simulink library "LIB_TF_G_12_StepControl"  (Simulink 8.6)
settings: Solver=ode45  StartTime=0.0  StopTime=10.0  RelTol=1e-3
PreLoadFcn:
  | if exist('tl_preloadfcn','file'), tl_preloadfcn(gcs,402); end
PostLoadFcn:
  | if exist('tl_postloadfcn','file'), tl_postloadfcn(gcs,402); end
undefined symbols (not defined in the file): ddv, u2, u3
libraries: tllib x4, LIB_TF_G_12_StepControl x1
(part 5 of 7)

== system LIB_TF_G_12_StepControl/TF_G_12_ManageEndingStep/Step execution in progress/ManageBeltPayOutAbortion/Belt Payout Abortion Opt Activated ==
  note: Belt Payout Interruption
  bBeltPayOutAbortion2 : Inport  RequirementInfo={} %GIDa_c23c1519_ce77_4f0e_84e0_58e9ce6e7015
  bBeltPayOutAbortion1 : Inport  RequirementInfo={} %GIDa_65d5ef8b_71e9_4e52_9127_813aec9379ea  Port=2
  u16BeltPayOutFiltered_mm : Inport  RequirementInfo={} %GIDa_03e05a97_4a46_4a00_a943_78f19d364a7f  Port=3
  Action Port : ActionPort  RequirementInfo={} %GIDa_ed5b74e4_286f_4c4b_a0da_10247e3268a9
  Constant3 : Constant  RequirementInfo={} %GIDa_df278d9b_a5ca_4067_b82a_a721af7a99c6  Value=ddv('BFE_Config_Data/CAL_KU16_BELT_PAYOUT_ABORTION_THRS1')  OutDataTypeStr=uint16  mask(TL_Constant){data={'output',{'variable','BFE_Config_Data/CAL_KU16_BELT_PAYOUT_ABORTION_THRS1'},'autoscaling',{'mode',2,'scalingvalid',1},'date',735951.66847480321}}
      settings: CopyFcn=if exist('tl_reset_reviewflag','file')==2,tl_reset_reviewflag(gcbh);end  DeleteFcn=if exist('delete_tlblock','file')==2,delete_tlblock(gcbh);end  NameChangeFcn=if exist('rename_tlblock','file')==2,rename_tlblock(gcbh);end  OpenFcn=if exist('tl_open_blockdlg','file')==2,tl_open_blockdlg(gcbh);else,open_system(gcbh,'parameter');end
      mask Help: eval(['if exist(''tl_online_help'',''file'') == 2, tl_online_help(''Topic'',''TL_Constant''),else, web([''jar:file:///'',matlabroot,''/help/toolbox/simulink/help.jar!/slref/' lower(get_param(gcbh,'Blocktype')) '.html''], ''-helpbrowser''),end'])
      mask Display: plot([-0.05, 1.05, NaN, -0.05, 1.05],[.01, .01, NaN, .99, .99])
  Constant5 : Constant  RequirementInfo={} %GIDa_6b8f2a3b_36a6_49af_a030_774c3046518c  Value=ddv('BFE_Config_Data/CAL_KU16_BELT_PAYOUT_ABORTION_THRS2')  OutDataTypeStr=uint16  mask(TL_Constant){data={'output',{'variable','BFE_Config_Data/CAL_KU16_BELT_PAYOUT_ABORTION_THRS2'},'autoscaling',{'mode',2,'scalingvalid',1},'date',735951.66847444442}}
      settings: CopyFcn=if exist('tl_reset_reviewflag','file')==2,tl_reset_reviewflag(gcbh);end  DeleteFcn=if exist('delete_tlblock','file')==2,delete_tlblock(gcbh);end  NameChangeFcn=if exist('rename_tlblock','file')==2,rename_tlblock(gcbh);end  OpenFcn=if exist('tl_open_blockdlg','file')==2,tl_open_blockdlg(gcbh);else,open_system(gcbh,'parameter');end
      mask Help: eval(['if exist(''tl_online_help'',''file'') == 2, tl_online_help(''Topic'',''TL_Constant''),else, web([''jar:file:///'',matlabroot,''/help/toolbox/simulink/help.jar!/slref/' lower(get_param(gcbh,'Blocktype')) '.html''], ''-helpbrowser''),end'])
      mask Display: plot([-0.05, 1.05, NaN, -0.05, 1.05],[.01, .01, NaN, .99, .99])
  Relational Operator1 : RelationalOperator  RequirementInfo={} %GIDa_2e279048_a574_4730_af74_afcb5488e17b  Operator=<=  OutDataTypeStr=boolean  mask(TL_RelationalOperator){data={'date',735951.6684740741}}
      settings: DeleteFcn=if exist('delete_tlblock','file')==2,delete_tlblock(gcbh);end  NameChangeFcn=if exist('rename_tlblock','file')==2,rename_tlblock(gcbh);end  OpenFcn=if exist('tl_open_blockdlg','file')==2,tl_open_blockdlg(gcbh);else,open_system(gcbh,'parameter');end
      mask Help: eval(['if exist(''tl_online_help'',''file'') == 2, tl_online_help(''Topic'',''TL_RelationalOperator''),else, web([''jar:file:///'',matlabroot,''/help/toolbox/simulink/help.jar!/slref/' lower(get_param(gcbh,'Blocktype')) '.html''], ''-helpbrowser''),end'])
      mask Display: plot([-0.05, 1.05, NaN, -0.05, 1.05],[.01, .01, NaN, .99, .99])
  Relational Operator2 : RelationalOperator  RequirementInfo={} %GIDa_1c9f918a_1d2a_4c1b_b35b_2dc0061f631d  OutDataTypeStr=boolean  mask(TL_RelationalOperator){data={'date',735951.66847383103}}
      settings: DeleteFcn=if exist('delete_tlblock','file')==2,delete_tlblock(gcbh);end  NameChangeFcn=if exist('rename_tlblock','file')==2,rename_tlblock(gcbh);end  OpenFcn=if exist('tl_open_blockdlg','file')==2,tl_open_blockdlg(gcbh);else,open_system(gcbh,'parameter');end
      mask Help: eval(['if exist(''tl_online_help'',''file'') == 2, tl_online_help(''Topic'',''TL_RelationalOperator''),else, web([''jar:file:///'',matlabroot,''/help/toolbox/simulink/help.jar!/slref/' lower(get_param(gcbh,'Blocktype')) '.html''], ''-helpbrowser''),end'])
      mask Display: plot([-0.05, 1.05, NaN, -0.05, 1.05],[.01, .01, NaN, .99, .99])
  anyBeltPayOutEvent : Logic  RequirementInfo="{'linktype_rmi_doors' '0000eac7 (/106886 BMW BMW L7 EL ECU PP R-EVAS-EMA_Phase_0/30_PRO_Requirements/Specification/05 Product Requirements/01 Main Functions/04_MF-04_To_Park_The_Belt_When_It_Is_Not_Fastened)' '#180' 'true' '2.3.2.1.1.0-19 Step 3:\t Abort step 3 (and go to Step 4) as soon as the belt ' ' ' ; 'linktype_rmi_doors' '0000eac7 (/106886 BMW BMW L7 EL ECU PP R-EVAS-EMA_Phase_0/30_PRO_Requirements/Specification/05 Product Requirements/01 Main Functions/04_MF-04_To_Park_The_Belt_When_It_Is_Not_Fastened)' '#186' 'true' '2.3.2.1.1.0-24 Step 5:\t Abort step 5 (and go to Step 6) as soon as the belt ' ' ' ; 'linktype_rmi_doors' '0000eac7 (/106886 BMW BMW L7 EL ECU PP R-EVAS-EMA_Phase_0/30_PRO_Requirements/Specification/05 Product Requirements/01 Main Functions/04_MF-04_To_Park_The_Belt_When_It_Is_Not_Fastened)' '#219' 'true' '2.3.2.2.1.0-19 Step 3:\t Abort step 3 (and go to Step 4) as soon as the belt ' '' ; 'linktype_rmi_doors' '0000eac7 (/106886 BMW BMW L7 EL ECU PP R-EVAS-EMA_Phase_0/30_PRO_Requirements/Specification/05 Product Requirements/01 Main Functions/04_MF-04_To_Park_The_Belt_When_It_Is_Not_Fastened)' '#224' 'true' '2.3.2.2.1.0-24 Step 5:\t Abort step 5 (and go to Step 6) as soon as the belt ' '' ; 'linktype_rmi_doors' '0000eac7 (/106886 BMW BMW L7 EL ECU PP R-EVAS-EMA_Phase_0/30_PRO_Requirements/Specification/05 Product Requirements/01 Main Functions/04_MF-04_To_Park_The_Belt_When_It_Is_Not_Fastened)' '#466' 'true' '2.4.4.2.1.2 Belt Payout' ' ' ; 'linktype_rmi_doors' '0000eac7 (/106886 BMW BMW L7 EL ECU PP R-EVAS-EMA_Phase_0/30_PRO_Requirements/Specification/05 Product Requirements/01 Main Functions/04_MF-04_To_Park_The_Belt_When_It_Is_Not_Fastened)' '#829' 'true' '2.4.4.2.1.2.1 High threshold' ' ' ; 'linktype_rmi_doors' '0000eac7 (/106886 BMW BMW L7 EL ECU PP R-EVAS-EMA_Phase_0/30_PRO_Requirements/Specification/05 Product Requirements/01 Main Functions/04_MF-04_To_Park_The_Belt_When_It_Is_Not_Fastened)' '#831' 'true' '2.4.4.2.1.2.1.0-1 Definition: Used to specify the minimum value of the belt pos' '' ; 'linktype_rmi_doors' '0000eac7 (/106886 BMW BMW L7 EL ECU PP R-EVAS-EMA_Phase_0/30_PRO_Requirements/Specification/05 Product Requirements/01 Main Functions/04_MF-04_To_Park_The_Belt_When_It_Is_Not_Fastened)' '#832' 'true' '2.4.4.2.1.2.1.0-2 Name: u16NvmHiBeltPayoutAbortThrs' ' ' ; 'linktype_rmi_doors' '0000eac7 (/106886 BMW BMW L7 EL ECU PP R-EVAS-EMA_Phase_0/30_PRO_Requirements/Specification/05 Product Requirements/01 Main Functions/04_MF-04_To_Park_The_Belt_When_It_Is_Not_Fastened)' '#833' 'true' '2.4.4.2.1.2.1.0-3 Type: SAFETY SOFTWARE' '' ; 'linktype_rmi_doors' '0000eac7 (/106886 BMW BMW L7 EL ECU PP R-EVAS-EMA_Phase_0/30_PRO_Requirements/Specification/05 Product Requirements/01 Main Functions/04_MF-04_To_Park_The_Belt_When_It_Is_Not_Fastened)' '#834' 'true' '2.4.4.2.1.2.1.0-4 Size: 2 bytes' '' ; 'linktype_rmi_doors' '0000eac7 (/106886 BMW BMW L7 EL ECU PP R-EVAS-EMA_Phase_0/30_PRO_Requirements/Specification/05 Product Requirements/01 Main Functions/04_MF-04_To_Park_The_Belt_When_It_Is_Not_Fastened)' '#835' 'true' '2.4.4.2.1.2.1.0-5 Scaling: 1LSB = 1mm' '' ; 'linktype_rmi_doors' '0000eac7 (/106886 BMW BMW L7 EL ECU PP R-EVAS-EMA_Phase_0/30_PRO_Requirements/Specification/05 Product Requirements/01 Main Functions/04_MF-04_To_Park_The_Belt_When_It_Is_Not_Fastened)' '#836' 'true' '2.4.4.2.1.2.1.0-6 Constraints: Unsigned full range = [0 ; 65535] = [0mm ; 65535' '' ; 'linktype_rmi_doors' '0000eac7 (/106886 BMW BMW L7 EL ECU PP R-EVAS-EMA_Phase_0/30_PRO_Requirements/Specification/05 Product Requirements/01 Main Functions/04_MF-04_To_Park_The_Belt_When_It_Is_Not_Fastened)' '#837' 'true' '2.4.4.2.1.2.1.0-7 Default value: 0x02EE = 750mm' '' ; 'linktype_rmi_doors' '0000eac7 (/106886 BMW BMW L7 EL ECU PP R-EVAS-EMA_Phase_0/30_PRO_Requirements/Specification/05 Product Requirements/01 Main Functions/04_MF-04_To_Park_The_Belt_When_It_Is_Not_Fastened)' '#838' 'true' '2.4.4.2.1.2.1.0-8 Access in normal mode (out of diagnosis session): READ only' '' ; 'linktype_rmi_doors' '0000eac7 (/106886 BMW BMW L7 EL ECU PP R-EVAS-EMA_Phase_0/30_PRO_Requirements/Specification/05 Product Requirements/01 Main Functions/04_MF-04_To_Park_The_Belt_When_It_Is_Not_Fastened)' '#830' 'true' '2.4.4.2.1.2.2 Low threshold' ' ' ; 'linktype_rmi_doors' '0000eac7 (/106886 BMW BMW L7 EL ECU PP R-EVAS-EMA_Phase_0/30_PRO_Requirements/Specification/05 Product Requirements/01 Main Functions/04_MF-04_To_Park_The_Belt_When_It_Is_Not_Fastened)' '#839' 'true' '2.4.4.2.1.2.2.0-1 Definition: Used to specify the minimum value of the belt pos' '' ; 'linktype_rmi_doors' '0000eac7 (/106886 BMW BMW L7 EL ECU PP R-EVAS-EMA_Phase_0/30_PRO_Requirements/Specification/05 Product Requirements/01 Main Functions/04_MF-04_To_Park_The_Belt_When_It_Is_Not_Fastened)' '#840' 'true' '2.4.4.2.1.2.2.0-2 Name: u16NvmLowBeltPayoutAbortThrs' ' ' ; 'linktype_rmi_doors' '0000eac7 (/106886 BMW BMW L7 EL ECU PP R-EVAS-EMA_Phase_0/30_PRO_Requirements/Specification/05 Product Requirements/01 Main Functions/04_MF-04_To_Park_The_Belt_When_It_Is_Not_Fastened)' '#841' 'true' '2.4.4.2.1.2.2.0-3 Type: SAFETY SOFTWARE' '' ; 'linktype_rmi_doors' '0000eac7 (/106886 BMW BMW L7 EL ECU PP R-EVAS-EMA_Phase_0/30_PRO_Requirements/Specification/05 Product Requirements/01 Main Functions/04_MF-04_To_Park_The_Belt_When_It_Is_Not_Fastened)' '#842' 'true' '2.4.4.2.1.2.2.0-4 Size: 2 bytes' '' ; 'linktype_rmi_doors' '0000eac7 (/106886 BMW BMW L7 EL ECU PP R-EVAS-EMA_Phase_0/30_PRO_Requirements/Specification/05 Product Requirements/01 Main Functions/04_MF-04_To_Park_The_Belt_When_It_Is_Not_Fastened)' '#843' 'true' '2.4.4.2.1.2.2.0-5 Scaling: 1LSB = 1mm' '' ; 'linktype_rmi_doors' '0000eac7 (/106886 BMW BMW L7 EL ECU PP R-EVAS-EMA_Phase_0/30_PRO_Requirements/Specification/05 Product Requirements/01 Main Functions/04_MF-04_To_Park_The_Belt_When_It_Is_Not_Fastened)' '#844' 'true' '2.4.4.2.1.2.2.0-6 Constraints: Unsigned full range = [0 ; 65535] = [0mm ; 65535' '' ; 'linktype_rmi_doors' '0000eac7 (/106886 BMW BMW L7 EL ECU PP R-EVAS-EMA_Phase_0/30_PRO_Requirements/Specification/05 Product Requirements/01 Main Functions/04_MF-04_To_Park_The_Belt_When_It_Is_Not_Fastened)' '#845' 'true' '2.4.4.2.1.2.2.0-7 Default value: 0x012C = 300mm' '' ; 'linktype_rmi_doors' '0000eac7 (/106886 BMW BMW L7 EL ECU PP R-EVAS-EMA_Phase_0/30_PRO_Requirements/Specification/05 Product Requirements/01 Main Functions/04_MF-04_To_Park_The_Belt_When_It_Is_Not_Fastened)' '#846' 'true' '2.4.4.2.1.2.2.0-8 Access in normal mode (out of diagnosis session): READ only' ' ' } %GIDa_a8192212_6ba7_426f_b05f_69b939d358c2"  Operator=OR  AllPortsSameDT=off  OutDataTypeStr=boolean  mask(TL_LogicalOperator){data={'date',735951.66847358795}}
      settings: DeleteFcn=if exist('delete_tlblock','file')==2,delete_tlblock(gcbh);end  NameChangeFcn=if exist('rename_tlblock','file')==2,rename_tlblock(gcbh);end  OpenFcn=if exist('tl_open_blockdlg','file')==2,tl_open_blockdlg(gcbh);else,open_system(gcbh,'parameter');end
      mask Help: eval(['if exist(''tl_online_help'',''file'') == 2, tl_online_help(''Topic'',''TL_LogicalOperator''),else, web([''jar:file:///'',matlabroot,''/help/toolbox/simulink/help.jar!/slref/' lower(get_param(gcbh,'Blocktype')) '.html''], ''-helpbrowser''),end'])
      mask Display: plot([-0.05, 1.05, NaN, -0.05, 1.05],[.01, .01, NaN, .99, .99])
  bBeltPayoutStepOptionExclusiveSet : Logic  RequirementInfo={} %GIDa_2a375b25_5cfa_4ca7_9be7_2ef03136cf89  Operator=XOR  AllPortsSameDT=off  OutDataTypeStr=boolean  mask(TL_LogicalOperator){data={'comment',{'text',['COD_BFE_00001' char(10) 'PO bits are defined for the "Belt PayOut Controlled" constraint under the following configuration:' char(10) '- 00 : "Belt PayOut controlled" constraint is not used' char(10) '- 01 : Low threshold (u16NvmLowBeltPayoutAbortThrs) is used' char(10) '- 10 : High threshold (u16NvmHiBeltPayoutAbortThrs) is used' char(10) '[COVERS : PRO_MF4_968]']},'output',{'name','$B'},'date',735951.66847333335}}
      settings: DeleteFcn=if exist('delete_tlblock','file')==2,delete_tlblock(gcbh);end  NameChangeFcn=if exist('rename_tlblock','file')==2,rename_tlblock(gcbh);end  OpenFcn=if exist('tl_open_blockdlg','file')==2,tl_open_blockdlg(gcbh);else,open_system(gcbh,'parameter');end
      mask Help: eval(['if exist(''tl_online_help'',''file'') == 2, tl_online_help(''Topic'',''TL_LogicalOperator''),else, web([''jar:file:///'',matlabroot,''/help/toolbox/simulink/help.jar!/slref/' lower(get_param(gcbh,'Blocktype')) '.html''], ''-helpbrowser''),end'])
      mask Display: plot([-0.05, 1.05, NaN, -0.05, 1.05],[.01, .01, NaN, .99, .99])
  u16NvmBeltPayoutAbortThrs1_Satisfy : Logic  RequirementInfo={} %GIDa_b2515d3c_dd19_480b_875b_9924ba5bbf92  Inputs=3  AllPortsSameDT=off  OutDataTypeStr=boolean  mask(TL_LogicalOperator){data={'date',735951.66847305559}}
      settings: DeleteFcn=if exist('delete_tlblock','file')==2,delete_tlblock(gcbh);end  NameChangeFcn=if exist('rename_tlblock','file')==2,rename_tlblock(gcbh);end  OpenFcn=if exist('tl_open_blockdlg','file')==2,tl_open_blockdlg(gcbh);else,open_system(gcbh,'parameter');end
      mask Help: eval(['if exist(''tl_online_help'',''file'') == 2, tl_online_help(''Topic'',''TL_LogicalOperator''),else, web([''jar:file:///'',matlabroot,''/help/toolbox/simulink/help.jar!/slref/' lower(get_param(gcbh,'Blocktype')) '.html''], ''-helpbrowser''),end'])
      mask Display: plot([-0.05, 1.05, NaN, -0.05, 1.05],[.01, .01, NaN, .99, .99])
  u16NvmBeltPayoutAbortThrs2_Satisfy : Logic  RequirementInfo={} %GIDa_f1047f13_8326_4e3c_a34e_0d6ae5728ff1  Inputs=3  AllPortsSameDT=off  OutDataTypeStr=boolean  mask(TL_LogicalOperator){data={'date',735951.66847275465}}
      settings: DeleteFcn=if exist('delete_tlblock','file')==2,delete_tlblock(gcbh);end  NameChangeFcn=if exist('rename_tlblock','file')==2,rename_tlblock(gcbh);end  OpenFcn=if exist('tl_open_blockdlg','file')==2,tl_open_blockdlg(gcbh);else,open_system(gcbh,'parameter');end
      mask Help: eval(['if exist(''tl_online_help'',''file'') == 2, tl_online_help(''Topic'',''TL_LogicalOperator''),else, web([''jar:file:///'',matlabroot,''/help/toolbox/simulink/help.jar!/slref/' lower(get_param(gcbh,'Blocktype')) '.html''], ''-helpbrowser''),end'])
      mask Display: plot([-0.05, 1.05, NaN, -0.05, 1.05],[.01, .01, NaN, .99, .99])
  bShallStepContinue : Outport  RequirementInfo={} %GIDa_64a204de_75df_4cc5_b6bd_1c3b809efabe
  wires:
  Relational Operator1/1 -> u16NvmBeltPayoutAbortThrs1_Satisfy/3
  Constant3/1 -> Relational Operator1/2
  Constant5/1 -> Relational Operator2/1
  Relational Operator2/1 -> u16NvmBeltPayoutAbortThrs2_Satisfy/1
  bBeltPayOutAbortion2/1 -> u16NvmBeltPayoutAbortThrs2_Satisfy/2, bBeltPayoutStepOptionExclusiveSet/1
  u16NvmBeltPayoutAbortThrs2_Satisfy/1 -> anyBeltPayOutEvent/1
  u16NvmBeltPayoutAbortThrs1_Satisfy/1 -> anyBeltPayOutEvent/2
  anyBeltPayOutEvent/1 -> bShallStepContinue/1
  u16BeltPayOutFiltered_mm/1 -> Relational Operator2/2, Relational Operator1/1
  bBeltPayoutStepOptionExclusiveSet/1 -> u16NvmBeltPayoutAbortThrs2_Satisfy/3, u16NvmBeltPayoutAbortThrs1_Satisfy/1
  bBeltPayOutAbortion1/1 -> u16NvmBeltPayoutAbortThrs1_Satisfy/2, bBeltPayoutStepOptionExclusiveSet/2

== system LIB_TF_G_12_StepControl/TF_G_12_ManageEndingStep/Step execution in progress/ManageBeltPayOutAbortion/Belt Payout Abortion Opt Deactivated ==
  Action Port : ActionPort  RequirementInfo={} %GIDa_c6f90e3b_f66f_4145_a0bd_dd5fd3e7edbc
  KB_FALSE : Constant  RequirementInfo={} %GIDa_fd22fdc3_6d5e_4ed9_8abf_b1b892869fac  Value=ddv('BFE/KB_FALSE')  OutDataTypeStr=boolean  SampleTime=-1  mask(TL_Constant){data={'output',{'variable','BFE/KB_FALSE'},'date',735951.66847248841}}
      settings: CopyFcn=if exist('tl_reset_reviewflag','file')==2,tl_reset_reviewflag(gcbh);end  DeleteFcn=if exist('delete_tlblock','file')==2,delete_tlblock(gcbh);end  NameChangeFcn=if exist('rename_tlblock','file')==2,rename_tlblock(gcbh);end  OpenFcn=if exist('tl_open_blockdlg','file')==2,tl_open_blockdlg(gcbh);else,open_system(gcbh,'parameter');end
      mask Help: eval(['if exist(''tl_online_help'',''file'') == 2, tl_online_help(''Topic'',''TL_Constant''),else, web([''jar:file:///'',matlabroot,''/help/toolbox/simulink/help.jar!/slref/' lower(get_param(gcbh,'Blocktype')) '.html''], ''-helpbrowser''),end'])
      mask Display: plot([-0.05, 1.05, NaN, -0.05, 1.05],[.01, .01, NaN, .99, .99])
  bShallStepContinue : Outport  RequirementInfo={} %GIDa_519f0a92_0f2a_43d0_80ad_a80812805cc2
  wires:
  KB_FALSE/1 -> bShallStepContinue/1

== system LIB_TF_G_12_StepControl/TF_G_12_ManageEndingStep/Step execution in progress/ManageMotorBlocked (Motor OverCurrent)/Motor Blocked Opt Activated ==
  u32MotorCurrent : Inport  RequirementInfo={} %GIDa_35077fa2_8525_40e9_ae14_395478e9e03d
  u16Temperature : Inport  RequirementInfo={} %GIDa_61ac1d77_d44d_43cd_babc_899375823a81  Port=2
  s16MotorPower : Inport  RequirementInfo={} %GIDa_1fed8ada_d606_4b4d_92f8_f6734bb26c11  Port=3
  u16BatteryVoltage : Inport  RequirementInfo={} %GIDa_ddfb933f_dae9_4570_b46d_68e419ca580a  Port=4
  bMotorBlockedControlled : Inport  RequirementInfo={} %GIDa_ae8f7be4_9352_48c1_9f9d_6020105d65ee  Port=5
  e_StepValidity Internal Status : Inport  RequirementInfo={} %GIDa_ddfb933f_dae9_4570_b46d_68e419ca580a  Port=6
  Action Port : ActionPort  RequirementInfo={} %GIDa_87bb87ed_56e9_449a_a862_c49058b79593
  If : If  RequirementInfo={} %GIDa_8d0784e2_3fab_4adf_9f81_7b4d294112bc  IfExpression=~u1
  If Action Subsystem : Subsystem  RequirementInfo={} %GIDa_865aa8e5_6704_479c_ad50_26c0c78900e7  TreatAsAtomicUnit=on
  If Action Subsystem1 : Subsystem  RequirementInfo={} %GIDa_8c5d38af_f00b_4300_b53e_cc8f71a37b7d  TreatAsAtomicUnit=on
  Merge : Merge  RequirementInfo={} %GIDa_e9bcc02d_e27f_4329_9329_51a7ee440049  mask(TL_Merge){data={'date',735951.66845872684}}
      settings: CopyFcn=if exist('tl_reset_reviewflag','file')==2,tl_reset_reviewflag(gcbh);end  DeleteFcn=if exist('delete_tlblock','file')==2,delete_tlblock(gcbh);end  NameChangeFcn=if exist('rename_tlblock','file')==2,rename_tlblock(gcbh);end  OpenFcn=if exist('tl_open_blockdlg','file')==2,tl_open_blockdlg(gcbh);else,open_system(gcbh,'parameter');end
      mask Help: eval(['if exist(''tl_online_help'',''file'') == 2, tl_online_help(''Topic'',''TL_Merge''),else, web([''jar:file:///'',matlabroot,''/help/toolbox/simulink/help.jar!/slref/' lower(get_param(gcbh,'Blocktype')) '.html''], ''-helpbrowser''),end'])
      mask Display: plot([-0.05, 1.05, NaN, -0.05, 1.05],[.01, .01, NaN, .99, .99])
  bInterruptStep : Outport  RequirementInfo={} %GIDa_c2568f75_19fb_49aa_9a96_6839ea089117
  wires:
  If/1 -> If Action Subsystem/Action
  bMotorBlockedControlled/1 -> If/1
  If/2 -> If Action Subsystem1/Action
  u32MotorCurrent/1 -> If Action Subsystem1/1(u32MotorCurrent)
  u16Temperature/1 -> If Action Subsystem1/2(u16Temperature)
  s16MotorPower/1 -> If Action Subsystem1/3(s16MotorPower)
  u16BatteryVoltage/1 -> If Action Subsystem1/4(u16BatteryVoltage)
  If Action Subsystem/1(bInterruptStep) -> Merge/1
  If Action Subsystem1/1(bInterruptStep) -> Merge/2
  Merge/1 -> bInterruptStep/1
  e_StepValidity Internal Status/1 -> If Action Subsystem1/5(e_StepValidity)

== system LIB_TF_G_12_StepControl/TF_G_12_ManageEndingStep/Step execution in progress/ManageMotorBlocked (Motor OverCurrent)/Motor Blocked Opt Deactivated ==
  Action Port : ActionPort  RequirementInfo={} %GIDa_c927e320_c65f_4372_9111_160f402852fa
  KB_FALSE : Constant  RequirementInfo={} %GIDa_fd272ef1_75ca_43bb_9878_25ed4256448c  Value=ddv('BFE/KB_FALSE')  OutDataTypeStr=boolean  SampleTime=-1  mask(TL_Constant){data={'output',{'variable','BFE/KB_FALSE'},'date',735951.66845836805}}
      settings: CopyFcn=if exist('tl_reset_reviewflag','file')==2,tl_reset_reviewflag(gcbh);end  DeleteFcn=if exist('delete_tlblock','file')==2,delete_tlblock(gcbh);end  NameChangeFcn=if exist('rename_tlblock','file')==2,rename_tlblock(gcbh);end  OpenFcn=if exist('tl_open_blockdlg','file')==2,tl_open_blockdlg(gcbh);else,open_system(gcbh,'parameter');end
      mask Help: eval(['if exist(''tl_online_help'',''file'') == 2, tl_online_help(''Topic'',''TL_Constant''),else, web([''jar:file:///'',matlabroot,''/help/toolbox/simulink/help.jar!/slref/' lower(get_param(gcbh,'Blocktype')) '.html''], ''-helpbrowser''),end'])
      mask Display: plot([-0.05, 1.05, NaN, -0.05, 1.05],[.01, .01, NaN, .99, .99])
  bInterruptStep : Outport  RequirementInfo={} %GIDa_46abf0d2_941a_4ccb_a280_e17c4bf6b063  InitialOutput=0
  wires:
  KB_FALSE/1 -> bInterruptStep/1

== system LIB_TF_G_12_StepControl/TF_G_12_ManageEndingStep/Step execution in progress/ManageTriggOff (end of holding steps)/TriggOff Opt Activated ==
  bTriggOffControlled : Inport  RequirementInfo={} %GIDa_cf12ec5b_9854_423e_a44e_6913c9bc66ab
  bIsNoMoreTensioningSituation : Inport  RequirementInfo={} %GIDa_3becb22c_9d79_4d7f_b005_4e906a452248  Port=2
  Action Port : ActionPort  RequirementInfo={} %GIDa_3b114ffe_8f83_495a_875f_317d4f567315
  B_TRUE : Constant  RequirementInfo={} %GIDa_b118b147_97b3_4247_834a_d341a382e0c8  Value=ddv('RTE_Define/KU8_TRUE')  OutDataTypeStr=uint8  SampleTime=-1  mask(TL_Constant){data={'output',{'variable','RTE_Define/KU8_TRUE'},'date',735951.66845699074}}
      settings: CopyFcn=if exist('tl_reset_reviewflag','file')==2,tl_reset_reviewflag(gcbh);end  DeleteFcn=if exist('delete_tlblock','file')==2,delete_tlblock(gcbh);end  NameChangeFcn=if exist('rename_tlblock','file')==2,rename_tlblock(gcbh);end  OpenFcn=if exist('tl_open_blockdlg','file')==2,tl_open_blockdlg(gcbh);else,open_system(gcbh,'parameter');end
      mask Help: eval(['if exist(''tl_online_help'',''file'') == 2, tl_online_help(''Topic'',''TL_Constant''),else, web([''jar:file:///'',matlabroot,''/help/toolbox/simulink/help.jar!/slref/' lower(get_param(gcbh,'Blocktype')) '.html''], ''-helpbrowser''),end'])
      mask Display: plot([-0.05, 1.05, NaN, -0.05, 1.05],[.01, .01, NaN, .99, .99])
  ManageTriggOff : Logic  RequirementInfo={} %GIDa_5649dccd_f0a5_450a_b266_b3777bd95ecf  AllPortsSameDT=off  OutDataTypeStr=boolean  mask(TL_LogicalOperator){data={'date',735951.66845665511}}
      settings: DeleteFcn=if exist('delete_tlblock','file')==2,delete_tlblock(gcbh);end  NameChangeFcn=if exist('rename_tlblock','file')==2,rename_tlblock(gcbh);end  OpenFcn=if exist('tl_open_blockdlg','file')==2,tl_open_blockdlg(gcbh);else,open_system(gcbh,'parameter');end
      mask Help: eval(['if exist(''tl_online_help'',''file'') == 2, tl_online_help(''Topic'',''TL_LogicalOperator''),else, web([''jar:file:///'',matlabroot,''/help/toolbox/simulink/help.jar!/slref/' lower(get_param(gcbh,'Blocktype')) '.html''], ''-helpbrowser''),end'])
      mask Display: plot([-0.05, 1.05, NaN, -0.05, 1.05],[.01, .01, NaN, .99, .99])
  RelationalOperator_bAccelerationLow : RelationalOperator  RequirementInfo={} %GIDa_26f27c81_779d_4171_a911_7f443c701b00  Operator===  OutDataTypeStr=boolean  mask(TL_RelationalOperator){data={'date',735951.66845641204}}
      settings: DeleteFcn=if exist('delete_tlblock','file')==2,delete_tlblock(gcbh);end  NameChangeFcn=if exist('rename_tlblock','file')==2,rename_tlblock(gcbh);end  OpenFcn=if exist('tl_open_blockdlg','file')==2,tl_open_blockdlg(gcbh);else,open_system(gcbh,'parameter');end
      mask Help: eval(['if exist(''tl_online_help'',''file'') == 2, tl_online_help(''Topic'',''TL_RelationalOperator''),else, web([''jar:file:///'',matlabroot,''/help/toolbox/simulink/help.jar!/slref/' lower(get_param(gcbh,'Blocktype')) '.html''], ''-helpbrowser''),end'])
      mask Display: plot([-0.05, 1.05, NaN, -0.05, 1.05],[.01, .01, NaN, .99, .99])
  bInterruptStep : Outport  RequirementInfo={} %GIDa_b6b92ec6_f112_4233_b8e9_8b9c41e8818c
  wires:
  RelationalOperator_bAccelerationLow/1 -> ManageTriggOff/2
  ManageTriggOff/1 -> bInterruptStep/1
  bTriggOffControlled/1 -> ManageTriggOff/1
  B_TRUE/1 -> RelationalOperator_bAccelerationLow/1
  bIsNoMoreTensioningSituation/1 -> RelationalOperator_bAccelerationLow/2

== system LIB_TF_G_12_StepControl/TF_G_12_ManageEndingStep/Step execution in progress/ManageTriggOff (end of holding steps)/TriggOff Opt Deactivated ==
  Action Port : ActionPort  RequirementInfo={} %GIDa_16121e16_5dbd_4791_9fa3_71739519c178
  KB_FALSE : Constant  RequirementInfo={} %GIDa_5f17e89d_8651_44bc_898e_efb4f55be7d3  Value=ddv('BFE/KB_FALSE')  OutDataTypeStr=boolean  SampleTime=-1  mask(TL_Constant){data={'output',{'variable','BFE/KB_FALSE'},'date',735951.66845615744}}
      settings: CopyFcn=if exist('tl_reset_reviewflag','file')==2,tl_reset_reviewflag(gcbh);end  DeleteFcn=if exist('delete_tlblock','file')==2,delete_tlblock(gcbh);end  NameChangeFcn=if exist('rename_tlblock','file')==2,rename_tlblock(gcbh);end  OpenFcn=if exist('tl_open_blockdlg','file')==2,tl_open_blockdlg(gcbh);else,open_system(gcbh,'parameter');end
      mask Help: eval(['if exist(''tl_online_help'',''file'') == 2, tl_online_help(''Topic'',''TL_Constant''),else, web([''jar:file:///'',matlabroot,''/help/toolbox/simulink/help.jar!/slref/' lower(get_param(gcbh,'Blocktype')) '.html''], ''-helpbrowser''),end'])
      mask Display: plot([-0.05, 1.05, NaN, -0.05, 1.05],[.01, .01, NaN, .99, .99])
  bInterruptStep : Outport  RequirementInfo={} %GIDa_a8bae8e5_6f65_4341_aed5_7f3de19c63f1  InitialOutput=0
  wires:
  KB_FALSE/1 -> bInterruptStep/1

== system LIB_TF_G_12_StepControl/TF_G_12_ControlStepExecution/New Step started/Adapt Step Target Value/Temperature Weighted/Step Order Negative ==
  u16_Temperature : Inport
  Action Port : ActionPort
  SelectReleasingFactor : Lookup_n-D  RequirementInfo={} %GIDa_47b51c6a_e422_47ae_b980_07d09d9204ea  NumberOfTableDimensions=1  BreakpointsForDimension1=ddv('BFE_Config_Data/CFG_au16TempWeightIndexRelease')  BreakpointsForDimension2=[1:3]  IndexSearchMethod=Linear search  Table=ddv('BFE_Config_Data/CFG_au8TempWeightFactorsRelease')  ExtrapMethod=Clip  OutDataTypeStr=uint8  InputSameDT=on  mask(TL_Lookup1D){data={'input',{'variable','BFE_Config_Data/CFG_au16TempWeightIndexRelease'},'output',{'type','UInt8'},'table',{'variable','BFE_Config_Data/CFG_au8TempWeightFactorsRelease'},'date',735951.66799130791}}
      settings: CopyFcn=if exist('tl_reset_reviewflag','file')==2,tl_reset_reviewflag(gcbh);end  DeleteFcn=if exist('delete_tlblock','file')==2,delete_tlblock(gcbh);end  NameChangeFcn=if exist('rename_tlblock','file')==2,rename_tlblock(gcbh);end  OpenFcn=if exist('tl_open_blockdlg','file')==2,tl_open_blockdlg(gcbh);else,open_system(gcbh,'parameter');end
      mask Help: eval(['if exist(''tl_online_help'',''file'') == 2, tl_online_help(''Topic'',''TL_Lookup1D''),else, web([''jar:file:///'',matlabroot,''/help/toolbox/simulink/help.jar!/slref/' lower(get_param(gcbh,'Blocktype')) '.html''], ''-helpbrowser''),end'])
      mask Display: plot([-0.05, 1.05, NaN, -0.05, 1.05],[.01, .01, NaN, .99, .99])
  Out1 : Outport  InitialOutput=64
  wires:
  SelectReleasingFactor/1 -> Out1/1
  u16_Temperature/1 -> SelectReleasingFactor/1

== system LIB_TF_G_12_StepControl/TF_G_12_ControlStepExecution/New Step started/Adapt Step Target Value/Temperature Weighted/Step Order Positive ==
  u16_Temperature : Inport
  e_TemperatureCompensationType : Inport  Port=2
  Action Port : ActionPort
  Data Type Conversion : DataTypeConversion
  Merge : Merge  Inputs=5  InitialOutput=64  mask(TL_Merge){data={'date',735951.66799019673}}
      settings: CopyFcn=if exist('tl_reset_reviewflag','file')==2,tl_reset_reviewflag(gcbh);end  DeleteFcn=if exist('delete_tlblock','file')==2,delete_tlblock(gcbh);end  NameChangeFcn=if exist('rename_tlblock','file')==2,rename_tlblock(gcbh);end  OpenFcn=if exist('tl_open_blockdlg','file')==2,tl_open_blockdlg(gcbh);else,open_system(gcbh,'parameter');end
      mask Help: eval(['if exist(''tl_online_help'',''file'') == 2, tl_online_help(''Topic'',''TL_Merge''),else, web([''jar:file:///'',matlabroot,''/help/toolbox/simulink/help.jar!/slref/' lower(get_param(gcbh,'Blocktype')) '.html''], ''-helpbrowser''),end'])
      mask Display: plot([-0.05, 1.05, NaN, -0.05, 1.05],[.01, .01, NaN, .99, .99])
  Switch Case : SwitchCase  CaseConditions={0,1,2,3}
  Switch Case Action Subsystem : Subsystem  TreatAsAtomicUnit=on
  Switch Case Action Subsystem1 : Subsystem  TreatAsAtomicUnit=on
  Switch Case Action Subsystem2 : Subsystem  TreatAsAtomicUnit=on
  Switch Case Action Subsystem3 : Subsystem  TreatAsAtomicUnit=on
  Switch Case Action Subsystem4 : Subsystem  TreatAsAtomicUnit=on
  Out1 : Outport  InitialOutput=64
  wires:
  Switch Case/1 -> Switch Case Action Subsystem/Action
  e_TemperatureCompensationType/1 -> Switch Case/1
  Switch Case/2 -> Switch Case Action Subsystem1/Action
  Switch Case/3 -> Switch Case Action Subsystem2/Action
  Switch Case/4 -> Switch Case Action Subsystem3/Action
  Switch Case/5 -> Switch Case Action Subsystem4/Action
  u16_Temperature/1 -> Switch Case Action Subsystem3/1(In1), Switch Case Action Subsystem2/1(In1), Switch Case Action Subsystem1/1(In1), Switch Case Action Subsystem/1(In1)
  Merge/1 -> Data Type Conversion/1
  Switch Case Action Subsystem/1(Out1) -> Merge/1
  Switch Case Action Subsystem1/1(Out1) -> Merge/2
  Switch Case Action Subsystem2/1(Out1) -> Merge/3
  Switch Case Action Subsystem3/1(Out1) -> Merge/4
  Switch Case Action Subsystem4/1(Out1) -> Merge/5
  Data Type Conversion/1 -> Out1/1

== system LIB_TF_G_12_StepControl/TF_G_12_ControlStepExecution/New Step started/Adapt Step Target Value/Temperature Weighted/Step Order equal 0 ==
  Action Port : ActionPort
  KU8_NO_WEIGHT : Constant  RequirementInfo={} %GIDa_e5136e51_baef_4cbd_8532_8a4a1a3d3f5e  Value=ddv('BFE/KUC_NEUTRAL_WEIGHT')  OutDataTypeStr=uint8  mask(TL_Constant){data={'output',{'variable','BFE/KUC_NEUTRAL_WEIGHT'},'date',735951.66798461811}}
      settings: CopyFcn=if exist('tl_reset_reviewflag','file')==2,tl_reset_reviewflag(gcbh);end  DeleteFcn=if exist('delete_tlblock','file')==2,delete_tlblock(gcbh);end  NameChangeFcn=if exist('rename_tlblock','file')==2,rename_tlblock(gcbh);end  OpenFcn=if exist('tl_open_blockdlg','file')==2,tl_open_blockdlg(gcbh);else,open_system(gcbh,'parameter');end
      mask Help: eval(['if exist(''tl_online_help'',''file'') == 2, tl_online_help(''Topic'',''TL_Constant''),else, web([''jar:file:///'',matlabroot,''/help/toolbox/simulink/help.jar!/slref/' lower(get_param(gcbh,'Blocktype')) '.html''], ''-helpbrowser''),end'])
      mask Display: plot([-0.05, 1.05, NaN, -0.05, 1.05],[.01, .01, NaN, .99, .99])
  Out1 : Outport  InitialOutput=64
  wires:
  KU8_NO_WEIGHT/1 -> Out1/1

== system LIB_TF_G_12_StepControl/TF_G_12_ControlStepExecution/New Step started/AdaptOrderType/If Action Subsystem/If Action Subsystem ==
  Action Port : ActionPort  RequirementInfo={} %GIDa_c2be52a6_334d_4efe_8787_d3b3e6b7d6cc
  High Power Config Preprocessor : Constant  RequirementInfo={} %GIDa_a84f456e_23de_481a_9bc2_f4fd956aa8ee  SampleTime=-1  mask(TL_Constant){data={'output',{'variable','BFE_Config_PreProc/BFE_CFG_OPT_HIGH_POWER'},'date',735951.6679834954}}
      settings: CopyFcn=if exist('tl_reset_reviewflag','file')==2,tl_reset_reviewflag(gcbh);end  DeleteFcn=if exist('delete_tlblock','file')==2,delete_tlblock(gcbh);end  NameChangeFcn=if exist('rename_tlblock','file')==2,rename_tlblock(gcbh);end  OpenFcn=if exist('tl_open_blockdlg','file')==2,tl_open_blockdlg(gcbh);else,open_system(gcbh,'parameter');end
      mask Help: eval(['if exist(''tl_online_help'',''file'') == 2, tl_online_help(''Topic'',''TL_Constant''),else, web([''jar:file:///'',matlabroot,''/help/toolbox/simulink/help.jar!/slref/' lower(get_param(gcbh,'Blocktype')) '.html''], ''-helpbrowser''),end'])
      mask Display: plot([-0.05, 1.05, NaN, -0.05, 1.05],[.01, .01, NaN, .99, .99])
  If Action Subsystem : Subsystem  TreatAsAtomicUnit=on
  If Action Subsystem1 : Subsystem  TreatAsAtomicUnit=on
  Merge : Merge  mask(TL_Merge){data={'date',735951.66798236116}}
      settings: CopyFcn=if exist('tl_reset_reviewflag','file')==2,tl_reset_reviewflag(gcbh);end  DeleteFcn=if exist('delete_tlblock','file')==2,delete_tlblock(gcbh);end  NameChangeFcn=if exist('rename_tlblock','file')==2,rename_tlblock(gcbh);end  OpenFcn=if exist('tl_open_blockdlg','file')==2,tl_open_blockdlg(gcbh);else,open_system(gcbh,'parameter');end
      mask Help: eval(['if exist(''tl_online_help'',''file'') == 2, tl_online_help(''Topic'',''TL_Merge''),else, web([''jar:file:///'',matlabroot,''/help/toolbox/simulink/help.jar!/slref/' lower(get_param(gcbh,'Blocktype')) '.html''], ''-helpbrowser''),end'])
      mask Display: plot([-0.05, 1.05, NaN, -0.05, 1.05],[.01, .01, NaN, .99, .99])
  Preprocessor IF : If  RequirementInfo={} %GIDa_74fcfe51_ce86_49e7_a8e3_74dd049d6189  IfExpression=u1  mask(TL_PreProcessorIf){data={'mode',2,'date',735951.66798203706}}
      settings: DeleteFcn=if exist('delete_tlblock','file')==2,delete_tlblock(gcbh);end  NameChangeFcn=if exist('rename_tlblock','file')==2,rename_tlblock(gcbh);end  OpenFcn=if exist('tl_open_blockdlg','file')==2,tl_open_blockdlg(gcbh);else,open_system(gcbh,'parameter');end
      mask Help: eval(['if exist(''tl_online_help'',''file'') == 2, tl_online_help(''Topic'',''TL_PreProcessorIf''),else, web([''jar:file:///'',matlabroot,''/help/toolbox/simulink/help.jar!/slref/' lower(get_param(gcbh,'Blocktype')) '.html''], ''-helpbrowser''),end'])
      mask Display:
      | plot([-0.05, 1.05, NaN, -0.05, 1.05],[.01, .01, NaN, .99, .99])
      | 
      | port_label('input', 1, 'u1')
      | port_label('output',1,'#ifdef u1');
      | port_label('output',2,'#else');
  Out1 : Outport  RequirementInfo={} %GIDa_b0c9ae98_6dba_45db_af28_83fd20c21001
  wires:
  High Power Config Preprocessor/1 -> Preprocessor IF/1
  Preprocessor IF/1 -> If Action Subsystem/Action
  Preprocessor IF/2 -> If Action Subsystem1/Action
  Merge/1 -> Out1/1
  If Action Subsystem/1(Out1) -> Merge/1
  If Action Subsystem1/1(Out1) -> Merge/2

== system LIB_TF_G_12_StepControl/TF_G_12_ControlStepExecution/New Step started/AdaptOrderType/If Action Subsystem/If Action Subsystem1 ==
  Action Port : ActionPort  RequirementInfo={} %GIDa_a6de8d00_e67b_40a1_a9ef_9a35133d2350
  If Action Subsystem : Subsystem  TreatAsAtomicUnit=on
  If Action Subsystem1 : Subsystem  TreatAsAtomicUnit=on
  Merge : Merge  mask(TL_Merge){data={'date',735951.6679810764}}
      settings: CopyFcn=if exist('tl_reset_reviewflag','file')==2,tl_reset_reviewflag(gcbh);end  DeleteFcn=if exist('delete_tlblock','file')==2,delete_tlblock(gcbh);end  NameChangeFcn=if exist('rename_tlblock','file')==2,rename_tlblock(gcbh);end  OpenFcn=if exist('tl_open_blockdlg','file')==2,tl_open_blockdlg(gcbh);else,open_system(gcbh,'parameter');end
      mask Help: eval(['if exist(''tl_online_help'',''file'') == 2, tl_online_help(''Topic'',''TL_Merge''),else, web([''jar:file:///'',matlabroot,''/help/toolbox/simulink/help.jar!/slref/' lower(get_param(gcbh,'Blocktype')) '.html''], ''-helpbrowser''),end'])
      mask Display: plot([-0.05, 1.05, NaN, -0.05, 1.05],[.01, .01, NaN, .99, .99])
  PID Config Preprocessor : Constant  RequirementInfo={} %GIDa_7eafd67b_d2ee_435e_a381_2faa064c9eec  SampleTime=-1  mask(TL_Constant){data={'output',{'variable','BFE_Config_PreProc/BFE_CFG_OPT_PID'},'date',735951.66798071761}}
      settings: CopyFcn=if exist('tl_reset_reviewflag','file')==2,tl_reset_reviewflag(gcbh);end  DeleteFcn=if exist('delete_tlblock','file')==2,delete_tlblock(gcbh);end  NameChangeFcn=if exist('rename_tlblock','file')==2,rename_tlblock(gcbh);end  OpenFcn=if exist('tl_open_blockdlg','file')==2,tl_open_blockdlg(gcbh);else,open_system(gcbh,'parameter');end
      mask Help: eval(['if exist(''tl_online_help'',''file'') == 2, tl_online_help(''Topic'',''TL_Constant''),else, web([''jar:file:///'',matlabroot,''/help/toolbox/simulink/help.jar!/slref/' lower(get_param(gcbh,'Blocktype')) '.html''], ''-helpbrowser''),end'])
      mask Display: plot([-0.05, 1.05, NaN, -0.05, 1.05],[.01, .01, NaN, .99, .99])
  Preprocessor IF : If  RequirementInfo={} %GIDa_3d3b2416_2ef2_4d02_9e3d_9e7d3b90d1a8  IfExpression=u1  mask(TL_PreProcessorIf){data={'mode',2,'date',735951.66798040504}}
      settings: DeleteFcn=if exist('delete_tlblock','file')==2,delete_tlblock(gcbh);end  NameChangeFcn=if exist('rename_tlblock','file')==2,rename_tlblock(gcbh);end  OpenFcn=if exist('tl_open_blockdlg','file')==2,tl_open_blockdlg(gcbh);else,open_system(gcbh,'parameter');end
      mask Help: eval(['if exist(''tl_online_help'',''file'') == 2, tl_online_help(''Topic'',''TL_PreProcessorIf''),else, web([''jar:file:///'',matlabroot,''/help/toolbox/simulink/help.jar!/slref/' lower(get_param(gcbh,'Blocktype')) '.html''], ''-helpbrowser''),end'])
      mask Display:
      | plot([-0.05, 1.05, NaN, -0.05, 1.05],[.01, .01, NaN, .99, .99])
      | 
      | port_label('input', 1, 'u1')
      | port_label('output',1,'#ifdef u1');
      | port_label('output',2,'#else');
  Out1 : Outport  RequirementInfo={} %GIDa_6ce8fbe6_8d9b_42e1_b25c_5a8739ef0574
  wires:
  PID Config Preprocessor/1 -> Preprocessor IF/1
  Preprocessor IF/1 -> If Action Subsystem/Action
  Preprocessor IF/2 -> If Action Subsystem1/Action
  If Action Subsystem/1(Out1) -> Merge/1
  If Action Subsystem1/1(Out1) -> Merge/2
  Merge/1 -> Out1/1

== system LIB_TF_G_12_StepControl/TF_G_12_ControlStepExecution/New Step started/AdaptOrderType/If Action Subsystem/If Action Subsystem2 ==
  Action Port : ActionPort  RequirementInfo={} %GIDa_98b51df9_2e8b_4cee_ae9d_f81abff0ab68
  If Action Subsystem : Subsystem  TreatAsAtomicUnit=on
  If Action Subsystem1 : Subsystem  TreatAsAtomicUnit=on
  Merge : Merge  mask(TL_Merge){data={'date',735951.66797946754}}
      settings: CopyFcn=if exist('tl_reset_reviewflag','file')==2,tl_reset_reviewflag(gcbh);end  DeleteFcn=if exist('delete_tlblock','file')==2,delete_tlblock(gcbh);end  NameChangeFcn=if exist('rename_tlblock','file')==2,rename_tlblock(gcbh);end  OpenFcn=if exist('tl_open_blockdlg','file')==2,tl_open_blockdlg(gcbh);else,open_system(gcbh,'parameter');end
      mask Help: eval(['if exist(''tl_online_help'',''file'') == 2, tl_online_help(''Topic'',''TL_Merge''),else, web([''jar:file:///'',matlabroot,''/help/toolbox/simulink/help.jar!/slref/' lower(get_param(gcbh,'Blocktype')) '.html''], ''-helpbrowser''),end'])
      mask Display: plot([-0.05, 1.05, NaN, -0.05, 1.05],[.01, .01, NaN, .99, .99])
  PID Config Preprocessor : Constant  RequirementInfo={} %GIDa_cc30653b_609b_4acf_8be2_dcff026115fb  SampleTime=-1  mask(TL_Constant){data={'output',{'variable','BFE_Config_PreProc/BFE_CFG_OPT_PID'},'date',735951.66797909723}}
      settings: CopyFcn=if exist('tl_reset_reviewflag','file')==2,tl_reset_reviewflag(gcbh);end  DeleteFcn=if exist('delete_tlblock','file')==2,delete_tlblock(gcbh);end  NameChangeFcn=if exist('rename_tlblock','file')==2,rename_tlblock(gcbh);end  OpenFcn=if exist('tl_open_blockdlg','file')==2,tl_open_blockdlg(gcbh);else,open_system(gcbh,'parameter');end
      mask Help: eval(['if exist(''tl_online_help'',''file'') == 2, tl_online_help(''Topic'',''TL_Constant''),else, web([''jar:file:///'',matlabroot,''/help/toolbox/simulink/help.jar!/slref/' lower(get_param(gcbh,'Blocktype')) '.html''], ''-helpbrowser''),end'])
      mask Display: plot([-0.05, 1.05, NaN, -0.05, 1.05],[.01, .01, NaN, .99, .99])
  Preprocessor IF : If  RequirementInfo={} %GIDa_b75425ed_b6f6_4f40_8043_084fbea54a18  IfExpression=u1  mask(TL_PreProcessorIf){data={'mode',2,'date',735951.66797878477}}
      settings: DeleteFcn=if exist('delete_tlblock','file')==2,delete_tlblock(gcbh);end  NameChangeFcn=if exist('rename_tlblock','file')==2,rename_tlblock(gcbh);end  OpenFcn=if exist('tl_open_blockdlg','file')==2,tl_open_blockdlg(gcbh);else,open_system(gcbh,'parameter');end
      mask Help: eval(['if exist(''tl_online_help'',''file'') == 2, tl_online_help(''Topic'',''TL_PreProcessorIf''),else, web([''jar:file:///'',matlabroot,''/help/toolbox/simulink/help.jar!/slref/' lower(get_param(gcbh,'Blocktype')) '.html''], ''-helpbrowser''),end'])
      mask Display:
      | plot([-0.05, 1.05, NaN, -0.05, 1.05],[.01, .01, NaN, .99, .99])
      | 
      | port_label('input', 1, 'u1')
      | port_label('output',1,'#ifdef u1');
      | port_label('output',2,'#else');
  Out1 : Outport  RequirementInfo={} %GIDa_ac0f761f_0166_4383_9e93_9abcc5b268c1
  wires:
  PID Config Preprocessor/1 -> Preprocessor IF/1
  Preprocessor IF/1 -> If Action Subsystem/Action
  Preprocessor IF/2 -> If Action Subsystem1/Action
  If Action Subsystem/1(Out1) -> Merge/1
  If Action Subsystem1/1(Out1) -> Merge/2
  Merge/1 -> Out1/1

== system LIB_TF_G_12_StepControl/TF_G_12_ControlStepExecution/New Step started/AdaptOrderType/If Action Subsystem/If Action Subsystem3 ==
  Action Port : ActionPort  RequirementInfo={} %GIDa_de3fd976_7fde_482f_a161_2e13ab1f763d
  KU8_CURRENT_STEP_TYPE : Constant  RequirementInfo={} %GIDa_d69a5c00_54f2_43d6_b971_f6dcd79dbea7  Value=ddv('BFE/Step_Def/KU8_CURRENT_STEP_TYPE')  OutDataTypeStr=uint8  mask(TL_Constant){data={'output',{'variable','BFE/Step_Def/KU8_CURRENT_STEP_TYPE'},'date',735951.66797859955}}
      settings: CopyFcn=if exist('tl_reset_reviewflag','file')==2,tl_reset_reviewflag(gcbh);end  DeleteFcn=if exist('delete_tlblock','file')==2,delete_tlblock(gcbh);end  NameChangeFcn=if exist('rename_tlblock','file')==2,rename_tlblock(gcbh);end  OpenFcn=if exist('tl_open_blockdlg','file')==2,tl_open_blockdlg(gcbh);else,open_system(gcbh,'parameter');end
      mask Help: eval(['if exist(''tl_online_help'',''file'') == 2, tl_online_help(''Topic'',''TL_Constant''),else, web([''jar:file:///'',matlabroot,''/help/toolbox/simulink/help.jar!/slref/' lower(get_param(gcbh,'Blocktype')) '.html''], ''-helpbrowser''),end'])
      mask Display: plot([-0.05, 1.05, NaN, -0.05, 1.05],[.01, .01, NaN, .99, .99])
  Out1 : Outport  RequirementInfo={} %GIDa_4ca8fdcf_657a_4017_b043_38228a29fcef  InitialOutput=1
  wires:
  KU8_CURRENT_STEP_TYPE/1 -> Out1/1

== system LIB_TF_G_12_StepControl/TF_G_12_ManageEndingStep/Step execution in progress/ManageMotorBlocked (Motor OverCurrent)/Motor Blocked Opt Activated/If Action Subsystem ==
  Action Port : ActionPort  RequirementInfo={} %GIDa_3a7e8853_e511_468c_991f_185d15d69cb6
  KB_FALSE : Constant  RequirementInfo={} %GIDa_33ee5824_cf63_440d_b205_e688adb6c057  Value=ddv('BFE/KB_FALSE')  OutDataTypeStr=boolean  SampleTime=-1  mask(TL_Constant){data={'output',{'variable','BFE/KB_FALSE'},'date',735951.66847050923}}
      settings: CopyFcn=if exist('tl_reset_reviewflag','file')==2,tl_reset_reviewflag(gcbh);end  DeleteFcn=if exist('delete_tlblock','file')==2,delete_tlblock(gcbh);end  NameChangeFcn=if exist('rename_tlblock','file')==2,rename_tlblock(gcbh);end  OpenFcn=if exist('tl_open_blockdlg','file')==2,tl_open_blockdlg(gcbh);else,open_system(gcbh,'parameter');end
      mask Help: eval(['if exist(''tl_online_help'',''file'') == 2, tl_online_help(''Topic'',''TL_Constant''),else, web([''jar:file:///'',matlabroot,''/help/toolbox/simulink/help.jar!/slref/' lower(get_param(gcbh,'Blocktype')) '.html''], ''-helpbrowser''),end'])
      mask Display: plot([-0.05, 1.05, NaN, -0.05, 1.05],[.01, .01, NaN, .99, .99])
  bInterruptStep : Outport  RequirementInfo={} %GIDa_313b6c61_8ed5_4ddc_870a_08c7fc37dea8  InitialOutput=0
  wires:
  KB_FALSE/1 -> bInterruptStep/1
